simulink model "eml_aero_radar"  (Simulink 7.6)
settings: Solver=ode5  SolverMode=SingleTasking  StartTime=0.0  StopTime=200  FixedStep=0.1  MaxStep=0.1  RelTol=1e-3  AbsTol=1e-6
PreLoadFcn:
  | aero_raddat;
undefined symbols (not defined in the file or in its folder): deltat, g, K, Speed, tauc, tauT
libraries: simulink x2, simulink_extras x1
CloseFcn:
  | h=findobj('type','figure');if ~isempty(h);close(h);end
settings Model: Creator=The MathWorks Inc.  CovMetricSettings=d  ExtModeTrigMode=oneshot  ExtModeArmWhenConnect=off  ExtModeAutoUpdateStatusClock=off
settings DataIOCC: LimitDataPoints=off  SaveOutput=off  TimeSaveName=t_sim  SignalLoggingName=logsOut
settings OptimizationCC: BlockReduction=off  BooleanDataType=off  InlineInvariantSignals=on  InitFltsAndDblsToZero=on  EfficientMapNaN2IntZero=off
settings DebuggingCC: SaveWithParameterizedLinksMsg=none  CheckExecutionContextPreStartOutputMsg=on  CheckExecutionContextRuntimeOutputMsg=on  SignalResolutionControl=TryResolveAllWithWarning  SolverPrmCheckMsg=none  MultiTaskDSMMsg=warning  MultiTaskCondExecSysMsg=none  StrictBusMsg=None
settings HardwareCC: TargetUnknown=on
settings SFSimCC: SimParseCustomCode=off
settings RTWCC: TemplateMakefile=grt_vc.tmf  IncludeERTFirstTime=on
settings CodeAppCC: MangleLength=5
settings GRTTargetCC: TargetFcnLib=ansi_tfl_tmw.mat

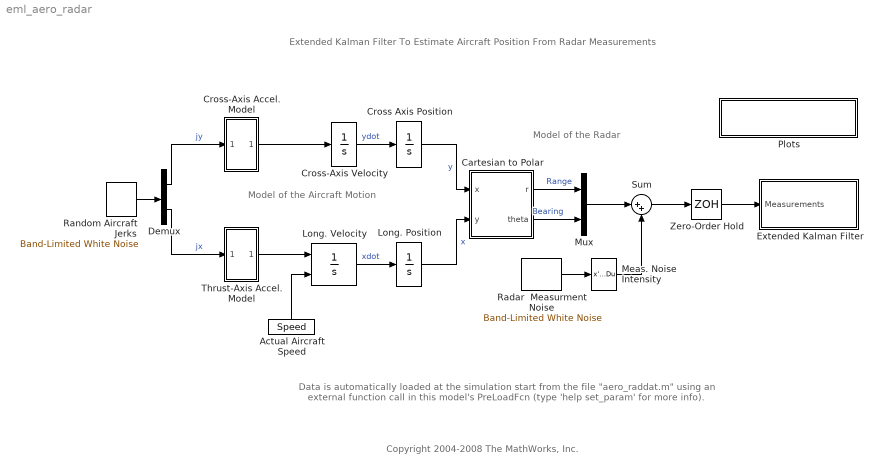
== system eml_aero_radar ==
  note: Data is automatically loaded at the simulation start from the file
      | "aero_raddat.m"
      | using an external function call in this model's PreLoadFcn
      | (type 'help set_param' for more info).
  note: Extended Kalman Filter To Estimate Aircraft Position From Radar Measurements
  note: Model of the Aircraft Motion
  note: Model of the Radar
  note: Copyright 2004-2008 The MathWorks, Inc.
  " Extended Kalman Filter" : Subsystem
  Actual Aircraft Speed : Constant  Value=Speed
  Cartesian to Polar : Subsystem
      mask Type: [x,y]->[r,theta]
      mask Description:
      | Tranformation from cartesian to polar
      | coordinates.
      | r=sqrt(x^2+y^2), theta=atan(y/x)
      mask Help: Unmask this block for more help.
      mask Display: plot(0,0,100,100,[24,20,15,20,20],[85,95,85,95,20],[80,20,95,85,95,85],[70,20,20,15,20,24],[56,56,55,52,50,46],[20,26,31,35,38,42])
  Cross Axis Position : Integrator
  Cross-Axis Accel. Model : Subsystem
  Cross-Axis Velocity : Integrator
  Demux : Demux  Outputs=2
  Long. Position : Integrator
  Long. Velocity : Integrator  InitialConditionSource=external
  Meas. Noise Intensity : StateSpace  A=[]  B=[]  C=[]  D=K  mask(Matrix Gain){K =[300 0; 0 .01]}
      mask prompts: K  "Gain matrix:"
      mask help: Matrix Gain.
      mask Help: Multiplies input vector by entered matrix to produce output vector (y=Au).
      mask Display: disp('K')
  Mux : Mux  Inputs=2
  Plots : Subsystem
      mask Display: disp('Plot Simulation Results')
  Radar  Measurment Noise : simulink/Sources/Band-Limited White Noise  SystemSampleTime=-1  Cov=[1 1]  Ts=0.1  seed=[52341 62341]
  Random Aircraft Jerks : simulink/Sources/Band-Limited White Noise  SystemSampleTime=-1  Cov=[0.004 .001]  Ts=0.1  seed=[12345 21343]
  Sum : Sum  Inputs=|++  SaturateOnIntegerOverflow=on  InputSameDT=on  OutDataTypeStr=Inherit: Same as first input
  Thrust-Axis Accel. Model : Subsystem
  Zero-Order Hold : ZeroOrderHold  SampleTime=deltat
  wires:
  Long. Position/1 -> Cartesian to Polar/2(y)  "x"
  Cartesian to Polar/2(theta) -> Mux/2  "Bearing"
  Cartesian to Polar/1(r) -> Mux/1  "Range"
  Mux/1 -> Sum/1
  Cross Axis Position/1 -> Cartesian to Polar/1(x)  "y"
  Cross-Axis Accel. Model/1(out_1) -> Cross-Axis Velocity/1
  Cross-Axis Velocity/1 -> Cross Axis Position/1  "ydot"
  Actual Aircraft Speed/1 -> Long. Velocity/2
  Long. Velocity/1 -> Long. Position/1  "xdot"
  Thrust-Axis Accel. Model/1(Acceleration) -> Long. Velocity/1
  Demux/1 -> Cross-Axis Accel. Model/1(Inport)  "jy"
  Demux/2 -> Thrust-Axis Accel. Model/1(Force)  "jx"
  Random Aircraft Jerks/1 -> Demux/1
  Radar  Measurment Noise/1 -> Meas. Noise Intensity/1
  Meas. Noise Intensity/1 -> Sum/2
  Sum/1 -> Zero-Order Hold/1
  Zero-Order Hold/1 -> " Extended Kalman Filter"/1(Measurements)

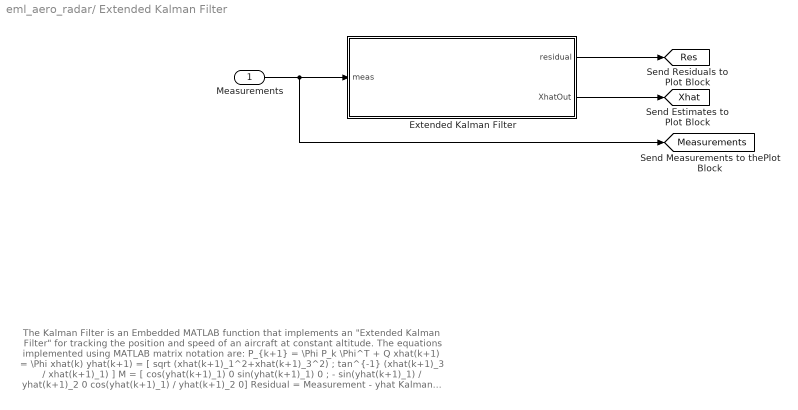
== system eml_aero_radar/ Extended Kalman Filter ==
  note: The Kalman Filter is an Embedded MATLAB function that implements an "Extended Kalman Filter" for tracking the
      | position and speed of an aircraft at constant altitude.  The equations implemented using MATLAB matrix notation are:
      |
      | P_{k+1} =  \Phi P_k \Phi^T + Q
      |
      | xhat(k+1) = \Phi xhat(k)
      |
      | yhat(k+1) = [  sqrt (xhat(k+1)_1^2+xhat(k+1)_3^2)  ; tan^{-1} (xhat(k+1)_3 / xhat(k+1)_1) ]
      |
      | M = [ cos(yhat(k+1)_1)  0 sin(yhat(k+1)_1)  0 ; - sin(yhat(k+1)_1) / yhat(k+1)_2  0  cos(yhat(k+1)_1) / yhat(k+1)_2  0]
      |
      | Residual = Measurement - yhat
      |
      | Kalman Gain:  W_{k+1} = P_{k+1} M^T (M P_{k+1} M^T + R)^{-1}
      |
      | xhat_{k+1} = xhat_{k+1} + W_{k+1} Residual
      |
      | P_{k+1} = ( I - W_{k+1} M ) P_{k+1}  ( I - W_{k+1} M ) ^T  + W_{k+1} R W_{k+1}^T
      |
      | Compare the Embedded MATLAB function with these equations.  You will see that there is a one-to-one correspondence.
  Measurements : Inport
  Extended Kalman Filter : Stateflow chart  TreatAsAtomicUnit=on
  tag scope: Measurements=global, Res=global, Xhat=global
  wires:
  Extended Kalman Filter/1(residual) -> [Res]
  Extended Kalman Filter/2(XhatOut) -> [Xhat]
  Measurements/1 -> Extended Kalman Filter/1(meas), [Measurements]

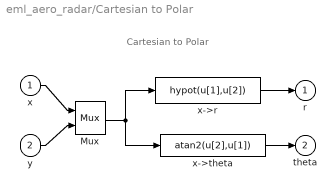
== system eml_aero_radar/Cartesian to Polar ==
  note: Cartesian to Polar
  x : Inport
  y : Inport  Port=2
  Mux : Mux  Inputs=2
  x->r : Fcn  Expr=hypot(u[1],u[2])
  x->theta : Fcn  Expr=atan2(u[2],u[1])
  r : Outport  InitialOutput=0
  theta : Outport  Port=2  InitialOutput=0
  wires:
  Mux/1 -> x->r/1, x->theta/1
  x->r/1 -> r/1
  x/1 -> Mux/1
  y/1 -> Mux/2
  x->theta/1 -> theta/1

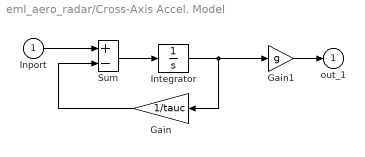
== system eml_aero_radar/Cross-Axis Accel. Model ==
  Inport : Inport
  Gain : Gain  Gain=1/tauc  SaturateOnIntegerOverflow=on  OutDataTypeStr=Inherit: Same as input  ParamDataTypeStr=Inherit: Same as input
  Gain1 : Gain  Gain=g  SaturateOnIntegerOverflow=on  OutDataTypeStr=Inherit: Same as input  ParamDataTypeStr=Inherit: Same as input
  Integrator : Integrator
  Sum : Sum  Inputs=+-  SaturateOnIntegerOverflow=on  InputSameDT=on  OutDataTypeStr=Inherit: Same as first input
  out_1 : Outport  InitialOutput=0
  wires:
  Inport/1 -> Sum/1
  Gain/1 -> Sum/2
  Integrator/1 -> Gain1/1, Gain/1
  Sum/1 -> Integrator/1
  Gain1/1 -> out_1/1

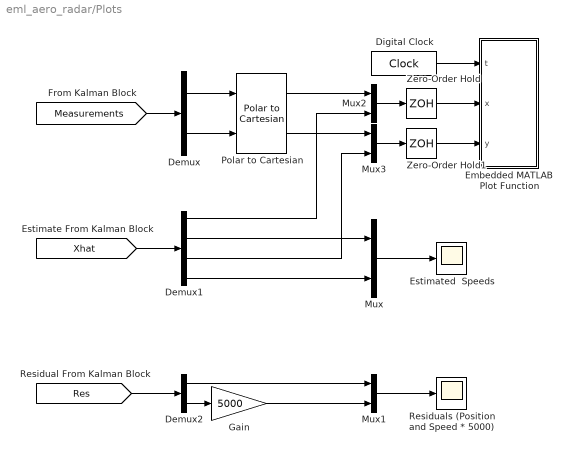
== system eml_aero_radar/Plots ==
  Demux : Demux  Outputs=2
  Demux1 : Demux
  Demux2 : Demux  Outputs=2
  Digital Clock : DigitalClock  SampleTime=deltat*5
  Embedded MATLAB Plot Function : Stateflow chart  TreatAsAtomicUnit=on
  Estimated  Speeds : Scope
      settings: TimeRange=200  YMin=-100  YMax=500
  Gain : Gain  Gain=5000
  Mux{,1..3} (4 alike) : Mux  Inputs=2
  Polar to Cartesian : simulink_extras/Transformations/Polar to Cartesian  SystemSampleTime=-1
  Residuals (Position and Speed * 5000) : Scope
      settings: TimeRange=200  YMin=-8000  YMax=6000
  Zero-Order Hold : ZeroOrderHold  SampleTime=deltat*2
  Zero-Order Hold1 : ZeroOrderHold  SampleTime=deltat*2
  wires:
  [Xhat] -> Demux1/1
  Demux1/1 -> Mux2/2
  Demux1/3 -> Mux3/2
  Demux1/2 -> Mux/1
  Demux1/4 -> Mux/2
  Mux/1 -> Estimated  Speeds/1
  [Measurements] -> Demux/1
  Demux/1 -> Polar to Cartesian/1
  Demux/2 -> Polar to Cartesian/2
  Polar to Cartesian/2 -> Mux3/1
  Polar to Cartesian/1 -> Mux2/1
  [Res] -> Demux2/1
  Demux2/2 -> Gain/1
  Demux2/1 -> Mux1/1
  Mux1/1 -> Residuals (Position and Speed * 5000)/1
  Gain/1 -> Mux1/2
  Mux2/1 -> Zero-Order Hold/1
  Mux3/1 -> Zero-Order Hold1/1
  Digital Clock/1 -> Embedded MATLAB Plot Function/1(t)
  Zero-Order Hold/1 -> Embedded MATLAB Plot Function/2(x)
  Zero-Order Hold1/1 -> Embedded MATLAB Plot Function/3(y)

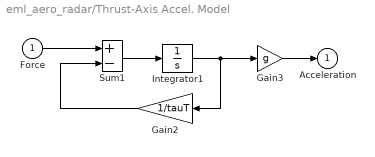
== system eml_aero_radar/Thrust-Axis Accel. Model ==
  Force : Inport
  Gain2 : Gain  Gain=1/tauT  SaturateOnIntegerOverflow=on  OutDataTypeStr=Inherit: Same as input  ParamDataTypeStr=Inherit: Same as input
  Gain3 : Gain  Gain=g  SaturateOnIntegerOverflow=on  OutDataTypeStr=Inherit: Same as input  ParamDataTypeStr=Inherit: Same as input
  Integrator1 : Integrator
  Sum1 : Sum  Inputs=+-  SaturateOnIntegerOverflow=on  InputSameDT=on  OutDataTypeStr=Inherit: Same as first input
  Acceleration : Outport  InitialOutput=0
  wires:
  Force/1 -> Sum1/1
  Gain2/1 -> Sum1/2
  Integrator1/1 -> Gain3/1, Gain2/1
  Sum1/1 -> Integrator1/1
  Gain3/1 -> Acceleration/1

== matlab function  Extended Kalman Filter/Extended Kalman Filter ==
  data: meas input double; residual output double; deltat parameter double; XhatOut output double
function [residual, XhatOut] = AERO_EXTKALMAN(meas, deltat)
%AERO_EXTKALMAN Radar Data Processing Tracker Using an Extended Kalman Filter
%
%  This program is executed as an embedded MATLAB function block in the 
%  aero_radmod Simulink model.  There is a file called "aero_raddat.m" that 
%  contains the data needed to run the eml_aero_radmod model.  The estimated 
%  and actual positions are plotted as the simulation runs using an additional 
%  embedded MATLAB function.
%
%  Compare the equations shown in the "eml_aero_radar/ Extended Kalman Filter"
%  subsystem, with the function shown below.

%  This program was developed by Dr. Richard Gran, September 1, 1996, 
%  and modified by Paul Barnard, June 1997. It was updated for inclusion 
%  as an Embedded MATLAB Function by Jason Ghidella, 2004
%  Copyright 1990-2004 The MathWorks, Inc.

    
%  Radar update time, deltat is a parameter, inherited from the workspace
%  where it was defined in the m-file aero_raddat.m

% Initialization

persistent P xhat

if isempty(P)
   P=zeros(4);
   xhat = [0.001 0.001 0 400]';
end

% 1. Compute Phi, Q, and R 
Phi = [1 deltat 0 0; 0 1 0 0 ; 0 0 1 deltat; 0 0 0 1];
Q =  diag([0 .005 0 .005]);
R =  diag([300^2 0.001^2]);

% 2. Propagate the covariance matrix:
P = Phi*P*Phi' + Q;

% 3. Propagate the track estimate:
xhat = Phi*xhat;

% 4 a). Compute observation estimates:
Rangehat = sqrt(xhat(1)^2+xhat(3)^2);
Bearinghat = atan2(xhat(3),xhat(1));

% 4 b). Compute observation vector y and linearized measurement matrix M 
yhat = 	[Rangehat;
         Bearinghat];
M = [ cos(Bearinghat)          0 sin(Bearinghat)          0
     -sin(Bearinghat)/Rangehat 0 cos(Bearinghat)/Rangehat 0 ];

% 4 c).  Compute residual (Estimation Error)
residual = meas - yhat;

% 5. Compute Kalman Gain:
W = P*M'*inv(M*P*M'+ R);

% 6. Update estimate
xhat = xhat + W*residual;

% 7. Update Covariance Matrix
P = (eye(4)-W*M)*P*(eye(4)-W*M)' + W*R*W';

XhatOut = xhat;

== matlab function Plots/Embedded MATLAB Plot Function ==
  data: t input double; x input double; y input double
function fcn(t,x,y)

eml.extrinsic('hold','clf','axis','plot','title','text','grid');

if t == 0
    hold('off'); clf;
    axis([-10000 30000 -10000 80000]); hold('on')
    plot([-10000 30000],[0 0])
    plot([0 0],[-10000 80000])
    title('\bf{Kalman Filter Using Embedded MATLAB}')
    text(-40000,-25000,'\rm\it{Position Measurements (Blue) & Position Estimates (Red)}')
    grid('on')
   
end
plot(x(1),y(1),'Marker','+','MarkerSize',3)
plot(x(2),y(2),'Marker','*','Color',[1 0 0],'MarkerSize',3)
